simulink model "Problem3_AutomaticTransmissionControl"  (R2020b)
settings: Solver=VariableStepAuto  StartTime=0.0  StopTime=10.0  RelTol=1e-3
values from neighbouring files (symbols this model uses):
  N20 = 0    [vehicleData.mat]
  Rfd = 3.23    [vehicleData.mat]
  rload0 = 40    [vehicleData.mat]
  rload2 = 0.3    [vehicleData.mat]
  Rw = 1    [vehicleData.mat]
undefined symbols (not defined in the file or in its folder): Iv
settings Model: DataDictionary=Data.sldd  Creator=vigne  LastModifiedBy=vigne

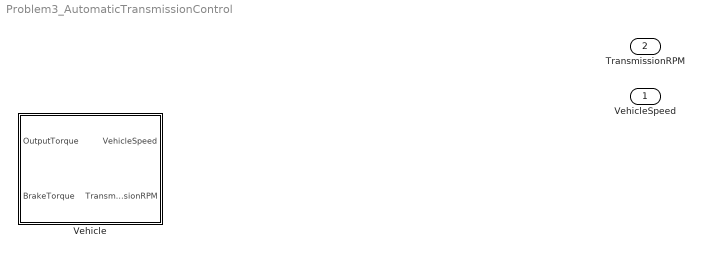
== system Problem3_AutomaticTransmissionControl ==
  Vehicle : Subsystem
  VehicleSpeed : Outport  Unit=mph  VectorParamsAs1DForOutWhenUnconnected=off
  TransmissionRPM : Outport  Port=2  Unit=rpm  VectorParamsAs1DForOutWhenUnconnected=off

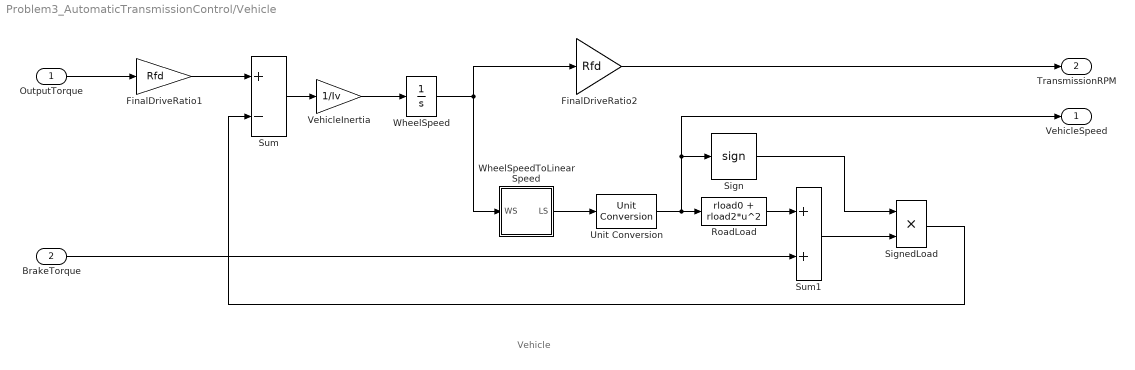
== system Problem3_AutomaticTransmissionControl/Vehicle ==
  note: Vehicle
  OutputTorque : Inport  Unit=ft*lbf@torque
  BrakeTorque : Inport  Port=2  Unit=ft*lbf@torque
  FinalDriveRatio1 : Gain  Gain=Rfd  SaturateOnIntegerOverflow=on  OutDataTypeStr=Inherit: Same as input  ParamDataTypeStr=Inherit: Same as input
  FinalDriveRatio2 : Gain  Gain=Rfd  SaturateOnIntegerOverflow=on  OutDataTypeStr=Inherit: Same as input  ParamDataTypeStr=Inherit: Same as input
  RoadLoad : Fcn  Expr=rload0 + rload2*u^2
  Sign : Signum
  SignedLoad : Product  InputSameDT=on  SaturateOnIntegerOverflow=on  OutDataTypeStr=Inherit: Same as first input
  Sum : Sum  Inputs=+-  InputSameDT=on  SaturateOnIntegerOverflow=on  OutDataTypeStr=Inherit: Same as first input
  Sum1 : Sum  InputSameDT=on  SaturateOnIntegerOverflow=on  OutDataTypeStr=Inherit: Same as first input
  Unit Conversion : UnitConversion
  VehicleInertia : Gain  Gain=1/Iv  SaturateOnIntegerOverflow=on  OutDataTypeStr=Inherit: Same as input  ParamDataTypeStr=Inherit: Same as input
  WheelSpeed : Integrator  InitialCondition=N20/Rfd  ZeroCross=off
  WheelSpeedToLinearSpeed : Subsystem
  VehicleSpeed : Outport  Unit=mph  VectorParamsAs1DForOutWhenUnconnected=off
  TransmissionRPM : Outport  Port=2  Unit=rpm  VectorParamsAs1DForOutWhenUnconnected=off
  wires:
  FinalDriveRatio2/1 -> TransmissionRPM/1
  Unit Conversion/1 -> VehicleSpeed/1, Sign/1, RoadLoad/1
  OutputTorque/1 -> FinalDriveRatio1/1
  Sum1/1 -> SignedLoad/2
  WheelSpeed/1 -> FinalDriveRatio2/1, WheelSpeedToLinearSpeed/1(WS)
  WheelSpeedToLinearSpeed/1(LS) -> Unit Conversion/1
  Sum/1 -> VehicleInertia/1
  Sign/1 -> SignedLoad/1
  BrakeTorque/1 -> Sum1/2
  SignedLoad/1 -> Sum/2
  RoadLoad/1 -> Sum1/1
  VehicleInertia/1 -> WheelSpeed/1
  FinalDriveRatio1/1 -> Sum/1

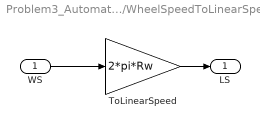
== system Problem3_AutomaticTransmissionControl/Vehicle/WheelSpeedToLinearSpeed ==
  WS : Inport  Unit=rpm
  ToLinearSpeed : Gain  Gain=2*pi*Rw  SaturateOnIntegerOverflow=on  OutDataTypeStr=Inherit: Same as input  ParamDataTypeStr=Inherit: Same as input
  LS : Outport  Unit=ft/min  VectorParamsAs1DForOutWhenUnconnected=off
  wires:
  ToLinearSpeed/1 -> LS/1
  WS/1 -> ToLinearSpeed/1
